simulink model "gazebo_cosimulation_simple_takeoff"  (R2023b)
settings: Solver=VariableStepAuto  StartTime=0.0  StopTime=10  RelTol=1e-3
undefined symbols (not defined in the file): center_cylinder, quadcopter, rotor_1, rotor_2, rotor_3, rotor_4
libraries: robotgazebolib x11, uavalgslib x1
settings Model: Creator=rakshan  LastModifiedBy=rakshan
settings DebuggingCC: ParameterPrecisionLossMsg=none

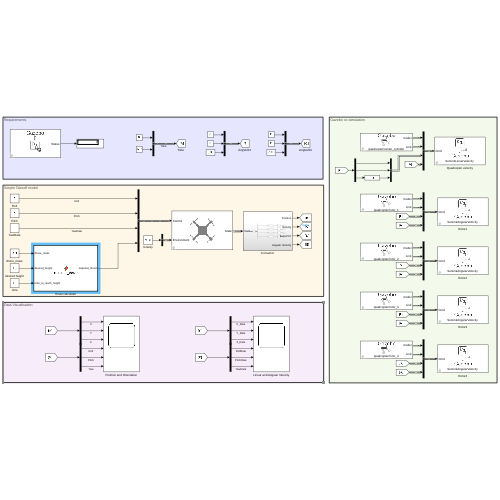
[thumbnail: Simulink's stored preview of the top-level diagram]
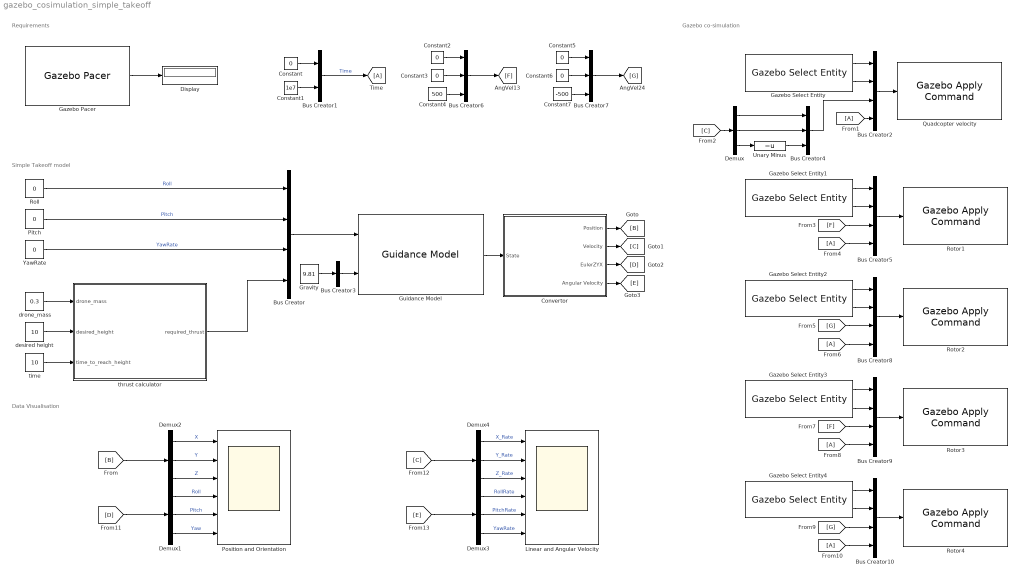
== system gazebo_cosimulation_simple_takeoff ==
  note: Data Visualisation
  note: Gazebo co-simulation
  note: Simple Takeoff model
  note: Requirements
  " time" : Constant  Value=10
  Bus Creator : BusCreator  Inputs=4  OutDataTypeStr=Bus: MultirotorGuidanceControlBus  NonVirtualBus=on
      settings: InheritFromInputs=off
  Bus Creator1 : BusCreator  Inputs=2  OutDataTypeStr=Bus: Gazebo_SL_Bus_gazebo_msgs_Time  NonVirtualBus=on
      settings: InheritFromInputs=off
  Bus Creator{5,8..10} (4 alike) : BusCreator  Inputs=4  OutDataTypeStr=Bus: Gazebo_SL_Bus_gazebo_msgs_SetLinkAngularVelocity  NonVirtualBus=on
      settings: InheritFromInputs=off
  Bus Creator2 : BusCreator  Inputs=4  OutDataTypeStr=Bus: Gazebo_SL_Bus_gazebo_msgs_SetLinkLinearVelocity  NonVirtualBus=on
      settings: InheritFromInputs=off
  Bus Creator3 : BusCreator  Inputs=1  OutDataTypeStr=Bus: MultirotorGuidanceEnvironmentBus  NonVirtualBus=on
      settings: InheritFromInputs=off
  Bus Creator4 : BusCreator  Inputs=3  OutDataTypeStr=Bus: Gazebo_SL_Bus_gazebo_msgs_Point  NonVirtualBus=on
      settings: InheritFromInputs=off
  Bus Creator6 : BusCreator  Inputs=3  OutDataTypeStr=Bus: Gazebo_SL_Bus_gazebo_msgs_Point  NonVirtualBus=on
      settings: InheritFromInputs=off
  Bus Creator7 : BusCreator  Inputs=3  OutDataTypeStr=Bus: Gazebo_SL_Bus_gazebo_msgs_Point  NonVirtualBus=on
      settings: InheritFromInputs=off
  Constant{,2..3,5..6} (5 alike) : Constant  Value=0
  Constant1 : Constant  Value=1e7
  Constant4 : Constant  Value=500
  Constant7 : Constant  Value=-500
  Convertor : Subsystem
  Demux{,1..4} (5 alike) : Demux  Outputs=3
  Display : Display
  From{1,4,6,8,10} (5 alike) : From
  Gazebo Pacer : robotgazebolib/Gazebo Pacer  ResetBehavior=Reset Gazebo simulation time  SampleTime=0.001
  Gazebo Select Entity : robotgazebolib/Gazebo Select Entity  modelElemName=quadcopter/center_cylinder  outputArraySize=128  OutputLabel=Link  SelectType=Link
  Gazebo Select Entity1 : robotgazebolib/Gazebo Select Entity  modelElemName=quadcopter/rotor_1  outputArraySize=128  OutputLabel=Link  SelectType=Link
  Gazebo Select Entity2 : robotgazebolib/Gazebo Select Entity  modelElemName=quadcopter/rotor_2  outputArraySize=128  OutputLabel=Link  SelectType=Link
  Gazebo Select Entity3 : robotgazebolib/Gazebo Select Entity  modelElemName=quadcopter/rotor_3  outputArraySize=128  OutputLabel=Link  SelectType=Link
  Gazebo Select Entity4 : robotgazebolib/Gazebo Select Entity  modelElemName=quadcopter/rotor_4  outputArraySize=128  OutputLabel=Link  SelectType=Link
  Gravity : Constant  Value=9.81
  Guidance Model : uavalgslib/Guidance Model  ModelType=MultirotorGuidance  SpecifiedDataType=double  SimulateUsing=Interpreted execution  InitialWorldPositionMultirotor=[0; 0; 0]  InitialWorldVelocityMultirotor=[0; 0; 0]  InitialEulerZYXMultirotor=[0; 0; 0]  InitialBodyAngularRateRPYMultirotor=[0; 0; 0]  InitialThrustMultirotor=0  InitialNorthFixedWing=0  InitialEastFixedWing=0  InitialHeightFixedWing=0  InitialAirSpeedFixedWing=0  InitialHeadingAngleFixedWing=0  InitialFlightPathAngleFixedWing=0  InitialRollAngleFixedWing=0  InitialRollAngleRateFixedWing=0  PDRollMultirotor=[3402.97,116.67]  PDPitchMultirotor=[3402.97, 116.67]  PYawRateMultirotor=1950  PThrustMultirotor=3900  MassMultirotor=0.3  PHeightFixedWing=3.9  PHeadingAngleFixedWing=3.9  PFlightPathAngleFixedWing=39  PDRollFixedWing=[3402.97, 116.67]  PAirSpeedFixedWing=1  FlightPathAngleLimitsFixedWing=[-pi/2, pi/2]  StateBusName='MultirotorGuidanceStateBus'  ControlBusName='MultirotorGuidanceControlBus'  EnvironmentBusName='MultirotorGuidanceEnvironmentBus'  DataType=double
  Linear and Angular Velocity : Scope  NumInputPorts=6
  Pitch : Constant  Value=0  OutDataTypeStr=double
  Position and Orientation : Scope  NumInputPorts=6
  Quadcopter velocity : robotgazebolib/Gazebo Apply Command  cmdType=SetLinkLinearVelocity  sampleTime=0.001
  Roll : Constant  Value=0  OutDataTypeStr=double
  Rotor{1..4} (4 alike) : robotgazebolib/Gazebo Apply Command  cmdType=SetLinkAngularVelocity  sampleTime=0.001
  Time : Goto
  Unary Minus : UnaryMinus
  YawRate : Constant  Value=0  OutDataTypeStr=double
  desired height : Constant  Value=10
  drone_mass : Constant  Value=0.3
  thrust calculator : MATLAB Function  TreatAsAtomicUnit=on
  wires:
  Pitch/1 -> Bus Creator/2  "Pitch"
  YawRate/1 -> Bus Creator/3  "YawRate"
  Roll/1 -> Bus Creator/1  "Roll"
  Bus Creator/1 -> Guidance Model/1
  Gravity/1 -> Bus Creator3/1
  Constant/1 -> Bus Creator1/1
  Constant1/1 -> Bus Creator1/2
  Bus Creator1/1 -> Time/1  "Time"
  Gazebo Select Entity/1 -> Bus Creator2/1
  Gazebo Select Entity/2 -> Bus Creator2/2
  Bus Creator2/1 -> Quadcopter velocity/1
  From1/1 -> Bus Creator2/4
  Bus Creator3/1 -> Guidance Model/2
  [C] -> Demux/1
  Demux/1 -> Bus Creator4/1
  Demux/2 -> Bus Creator4/2
  Demux/3 -> Unary Minus/1
  Bus Creator4/1 -> Bus Creator2/3
  Guidance Model/1 -> Convertor/1(State)
  Convertor/1(Position) -> [B]
  Convertor/2(Velocity) -> [C]
  Convertor/4(Angular Velocity) -> [E]
  Convertor/3(EulerZYX) -> [D]
  Unary Minus/1 -> Bus Creator4/3
  Gazebo Pacer/1 -> Display/1
  drone_mass/1 -> thrust calculator/1(drone_mass)
  desired height/1 -> thrust calculator/2(desired_height)
  " time"/1 -> thrust calculator/3(time_to_reach_height)
  thrust calculator/1(required_thrust) -> Bus Creator/4
  Bus Creator5/1 -> Rotor1/1
  Gazebo Select Entity1/1 -> Bus Creator5/1
  Gazebo Select Entity1/2 -> Bus Creator5/2
  Bus Creator6/1 -> [F]
  Constant2/1 -> Bus Creator6/1
  Constant3/1 -> Bus Creator6/2
  Constant4/1 -> Bus Creator6/3
  [F] -> Bus Creator5/3
  From4/1 -> Bus Creator5/4
  Constant7/1 -> Bus Creator7/3
  Constant6/1 -> Bus Creator7/2
  Constant5/1 -> Bus Creator7/1
  Bus Creator7/1 -> [G]
  From6/1 -> Bus Creator8/4
  [G] -> Bus Creator8/3
  Gazebo Select Entity2/2 -> Bus Creator8/2
  Gazebo Select Entity2/1 -> Bus Creator8/1
  Bus Creator8/1 -> Rotor2/1
  Bus Creator9/1 -> Rotor3/1
  Gazebo Select Entity3/1 -> Bus Creator9/1
  Gazebo Select Entity3/2 -> Bus Creator9/2
  [F] -> Bus Creator9/3
  From8/1 -> Bus Creator9/4
  From10/1 -> Bus Creator10/4
  [G] -> Bus Creator10/3
  Gazebo Select Entity4/2 -> Bus Creator10/2
  Gazebo Select Entity4/1 -> Bus Creator10/1
  Bus Creator10/1 -> Rotor4/1
  Demux1/1 -> Position and Orientation/4  "Roll"
  Demux1/2 -> Position and Orientation/5  "Pitch"
  Demux1/3 -> Position and Orientation/6  "Yaw"
  [D] -> Demux1/1
  Demux2/1 -> Position and Orientation/1  "X"
  Demux2/2 -> Position and Orientation/2  "Y"
  Demux2/3 -> Position and Orientation/3  "Z"
  [B] -> Demux2/1
  Demux4/1 -> Linear and Angular Velocity/1  "X_Rate"
  Demux3/2 -> Linear and Angular Velocity/5  "PitchRate"
  Demux3/3 -> Linear and Angular Velocity/6  "YawRate"
  [E] -> Demux3/1
  Demux4/3 -> Linear and Angular Velocity/3  "Z_Rate"
  Demux4/2 -> Linear and Angular Velocity/2  "Y_Rate"
  Demux3/1 -> Linear and Angular Velocity/4  "RollRate"
  [C] -> Demux4/1

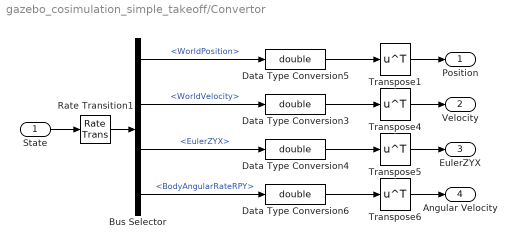
== system gazebo_cosimulation_simple_takeoff/Convertor ==
  State : Inport
  Bus Selector : BusSelector  OutputSignals=WorldPosition,WorldVelocity,EulerZYX,BodyAngularRateRPY
  Data Type Conversion{3..6} (4 alike) : DataTypeConversion  OutDataTypeStr=double  SaturateOnIntegerOverflow=off  RndMeth=Floor
  Rate Transition1 : RateTransition
  Transpose{1,4..6} (4 alike) : Math  Operator=transpose
  Position : Outport
  Velocity : Outport  Port=2
  EulerZYX : Outport  Port=3
  Angular Velocity : Outport  Port=4
  wires:
  Transpose5/1 -> EulerZYX/1
  Transpose4/1 -> Velocity/1
  Bus Selector/1 -> Data Type Conversion5/1  "<WorldPosition>"
  Bus Selector/4 -> Data Type Conversion6/1  "<BodyAngularRateRPY>"
  Transpose1/1 -> Position/1
  Bus Selector/3 -> Data Type Conversion4/1  "<EulerZYX>"
  Bus Selector/2 -> Data Type Conversion3/1  "<WorldVelocity>"
  Data Type Conversion4/1 -> Transpose5/1
  Data Type Conversion6/1 -> Transpose6/1
  Transpose6/1 -> Angular Velocity/1
  Data Type Conversion5/1 -> Transpose1/1
  Data Type Conversion3/1 -> Transpose4/1
  Rate Transition1/1 -> Bus Selector/1
  State/1 -> Rate Transition1/1

== matlab function gazebo_cosimulation_simple_takeoff/thrust calculator ==
  data: required_thrust output; drone_mass input; desired_height input; time_to_reach_height input
function required_thrust = calculate_thrust(drone_mass, desired_height, time_to_reach_height)
    % Constants
    g = 9.81;  % gravitational acceleration (m/s^2)
    
    % Calculate the required acceleration (assuming uniform acceleration)
    required_acceleration = 2 * desired_height / (time_to_reach_height ^ 2);
    
    % Total required thrust (mass * (g + required_acceleration))
    required_thrust = drone_mass * (g + required_acceleration);
end
